simulink model "second_loop"  (R2019b)
settings: Solver=VariableStepAuto  StartTime=0.0  StopTime=10.0  RelTol=1e-3
values from neighbouring files (symbols this model uses):
  K = [66.2259572254 -60.3086645892 5.93307364323 -20.4157003719]    [lqr_K.mat]    (also in lqr_controller.m = lqr(sys,Q,R); swmain.m = lqr_controller(sys2))
  sys = ss(A,B,C,D,-1)    [1b.m]    (also in get_system.m = ss(A,B,C,D); get_system2.m = ss(A,B,C,D); statespace.m = ss(A,B,C,D); swmain.m = get_system(params))
  x_d = desired_state(theta_d, params)    [swmain.m]
undefined symbols (not defined in the file or in its folder): Ts, wc
settings Model: Creator=martijndebeuf  LastModifiedBy=martijndebeuf

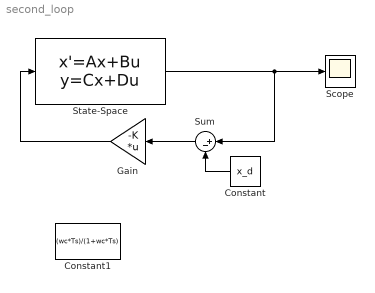
== system second_loop ==
  Constant : Constant  Value=x_d
  Constant1 : Constant  Value=(wc*Ts)/(1+wc*Ts)
  Gain : Gain  Gain=-K  Multiplication=Matrix(K*u) (u vector)
  Scope : Scope
  State-Space : StateSpace  A=sys.A  B=sys.B  C=eye(4)  D=zeros(4,1)  InitialCondition=initial_conditions'
  Sum : Sum  Inputs=|+-
  wires:
  Constant/1 -> Sum/2
  Sum/1 -> Gain/1
  State-Space/1 -> Sum/1, Scope/1
  Gain/1 -> State-Space/1
